simulink model "lab_8_1_unknown_input"  (R2023a)
settings: Solver=VariableStepAuto  StartTime=0.0  StopTime=10  RelTol=1e-3
values from neighbouring files (symbols this model uses):
  A = eye(3) + Ts * A    [part_deriv.m]
undefined symbols (not defined in the file or in its folder): Ae, B, Be, C, Ce, E, Ke, Le, x10, x20, x30
settings Model: Creator=bz  LastModifiedBy=bz

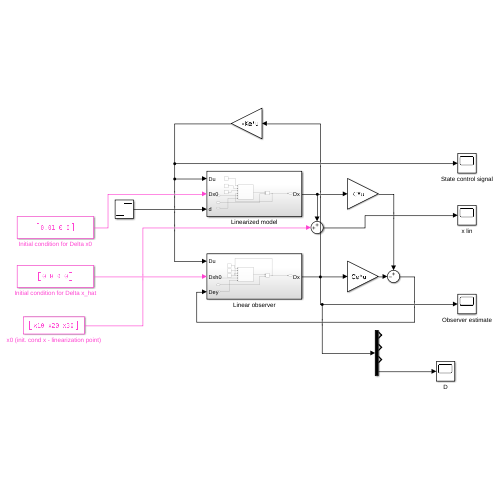
[thumbnail: Simulink's stored preview of the top-level diagram]
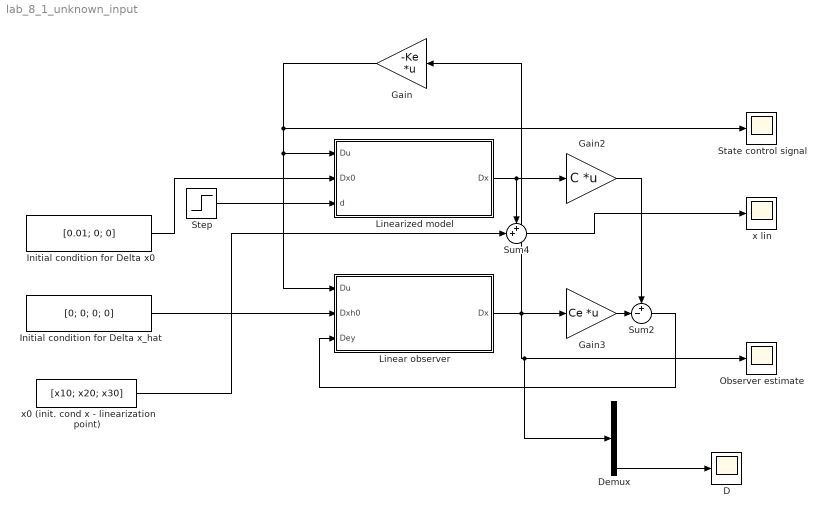
== system lab_8_1_unknown_input ==
  D : Scope
  Demux : Demux
  Gain : Gain  Gain=-Ke  Multiplication=Matrix(K*u)
  Gain2 : Gain  Gain=C  Multiplication=Matrix(K*u)
  Gain3 : Gain  Gain=Ce  Multiplication=Matrix(K*u)
  Initial condition for Delta x0 : Constant  Value=[0.01; 0; 0]
  Initial condition for Delta x_hat : Constant  Value=[0; 0; 0; 0]
  Linear observer : Subsystem
  Linearized model : Subsystem
  Observer estimate : Scope
  State control signal : Scope
  Step : Step  Time=3  SampleTime=0
  Sum2 : Sum  Inputs=+-|
  Sum4 : Sum  Inputs=++|
  x lin : Scope
  x0 (init. cond x - linearization point) : Constant  Value=[x10; x20; x30]
  wires:
  Initial condition for Delta x0/1 -> Linearized model/2(Dx0)
  x0 (init. cond x - linearization point)/1 -> Sum4/2
  Gain/1 -> State control signal/1, Linear observer/1(Du), Linearized model/1(Du)
  Linearized model/1(Dx) -> Gain2/1, Sum4/1
  Linear observer/1(Dx) -> Demux/1, Observer estimate/1, Gain3/1, Gain/1
  Initial condition for Delta x_hat/1 -> Linear observer/2(Dxh0)
  Sum2/1 -> Linear observer/3(Dey)
  Gain2/1 -> Sum2/1
  Gain3/1 -> Sum2/2
  Sum4/1 -> x lin/1
  Demux/4 -> D/1
  Step/1 -> Linearized model/3(d)

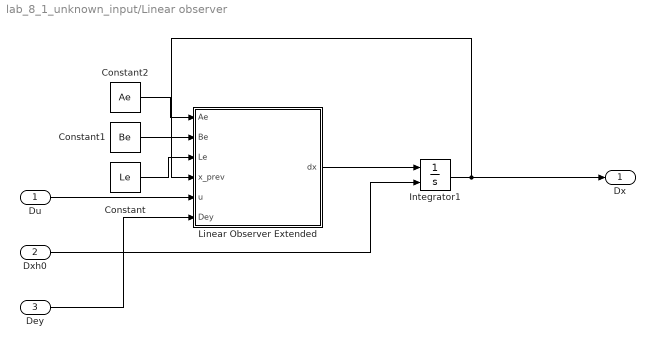
== system lab_8_1_unknown_input/Linear observer ==
  Du : Inport
  Dxh0 : Inport  Port=2
  Dey : Inport  Port=3
  Constant : Constant  Value=Le
  Constant1 : Constant  Value=Be
  Constant2 : Constant  Value=Ae
  Integrator1 : Integrator  InitialConditionSource=external
  Linear Observer Extended : MATLAB Function  TreatAsAtomicUnit=on
  Dx : Outport
  wires:
  Linear Observer Extended/1(dx) -> Integrator1/1
  Integrator1/1 -> Dx/1, Linear Observer Extended/4(x_prev)
  Dxh0/1 -> Integrator1/2
  Du/1 -> Linear Observer Extended/5(u)
  Dey/1 -> Linear Observer Extended/6(Dey)
  Constant/1 -> Linear Observer Extended/3(Le)
  Constant1/1 -> Linear Observer Extended/2(Be)
  Constant2/1 -> Linear Observer Extended/1(Ae)

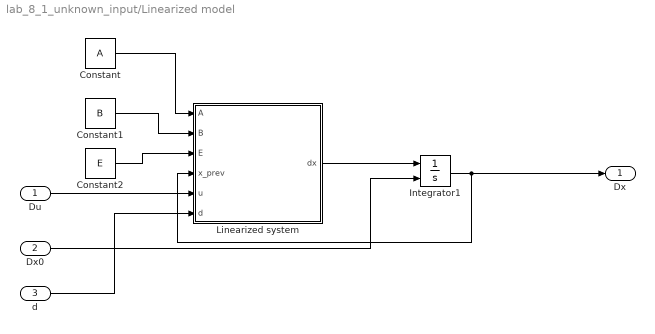
== system lab_8_1_unknown_input/Linearized model ==
  Du : Inport
  Dx0 : Inport  Port=2
  d : Inport  Port=3
  Constant : Constant  Value=A
  Constant1 : Constant  Value=B
  Constant2 : Constant  Value=E
  Integrator1 : Integrator  InitialConditionSource=external
  Linearized system : MATLAB Function  TreatAsAtomicUnit=on
  Dx : Outport
  wires:
  Linearized system/1(dx) -> Integrator1/1
  Integrator1/1 -> Dx/1, Linearized system/4(x_prev)
  Dx0/1 -> Integrator1/2
  Du/1 -> Linearized system/5(u)
  Constant/1 -> Linearized system/1(A)
  Constant1/1 -> Linearized system/2(B)
  Constant2/1 -> Linearized system/3(E)
  d/1 -> Linearized system/6(d)

== matlab function lab_8_1_unknown_input/Linearized model/Linearized system ==
  data: A input; B input; E input; x_prev input; u input; dx output size=[3,1]; d input
function dx = fcn(A, B, E, x_prev, u, d)

dx = A * x_prev + B * u + E * d;

end

== matlab function lab_8_1_unknown_input/Linear observer/Linear Observer Extended ==
  data: Ae input; Be input; Le input; x_prev input; u input; dx output; Dey input
function dx  = fcn(Ae, Be, Le, x_prev, u, Dey)

% x_prev

dx = Ae * x_prev + Be * u + Le * Dey;

end
